simulink model "YXPChFPID_jhua"  (Simulink 5.0)
settings: Solver=ode45  SolverMode=SingleTasking  StartTime=0.0  StopTime=1  FixedStep=0.001  RelTol=1e-3
settings Model: LastModifiedBy=ThinkPad  RTWOptions="-aEnforceIntegerDowncast=1 -aExtMode=0 -aExtModeTesting=0 -aFoldNonRolledExpr=1 -aForceParamTrailComments=0 -aGenerateComments=1 -aGenerateReport=0 -aIgnoreCustomStorageClasses=1 -aIncDataTypeInIds=0 -aIncHierarchyInIds=0 -aInlineInvariantSignals=0 -aInlinedPrmAccess=\"Literals\" -aLocalBlockOutputs=1 -aLogVarNameModifier=\"rt_\" -aMaxRTWIdLen=31 -aPrefixModelToSubsysFcnNames=1 -aRTWVerbose=1 -aRollThreshold=5 -aShowEliminatedStatements=0"

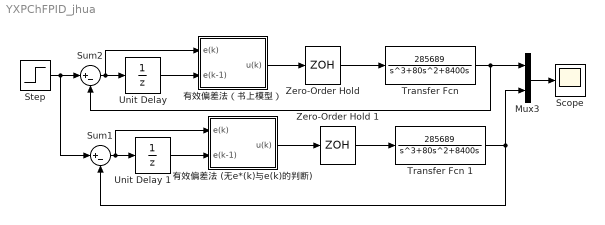
== system YXPChFPID_jhua ==
  "  Scope " : Scope
      settings: YMin=0  YMax=1.8  SaveName=YXPChFPIDI1  DataFormat=Array  MaxDataPoints=500000
  " Transfer Fcn " : TransferFcn  Numerator=[285689]  Denominator=[1 80 8400 0]
  " Transfer Fcn 1" : TransferFcn  Numerator=[285689]  Denominator=[1 80 8400 0]
  " Unit Delay " : UnitDelay  SampleTime=0.001
  " Unit Delay 1" : UnitDelay  SampleTime=0.001
  " Zero-Order Hold " : ZeroOrderHold  SampleTime=0.001
  " Zero-Order Hold 1" : ZeroOrderHold  SampleTime=0.001
  Mux3 : Mux  Inputs=2
  Step : Step  Time=0  After=30  SampleTime=0
  Sum1 : Sum  Inputs=|+-  SaturateOnIntegerOverflow=on
  Sum2 : Sum  Inputs=|+-  SaturateOnIntegerOverflow=on
  有效偏差法 (无e*(k)与e(k)的判断) : Subsystem
  有效偏差法（书上模型） : Subsystem
  wires:
  Step/1 -> Sum2/1, Sum1/1
  有效偏差法（书上模型）/1(u(k)) -> " Zero-Order Hold "/1
  " Zero-Order Hold "/1 -> " Transfer Fcn "/1
  " Transfer Fcn "/1 -> Sum2/2, Mux3/1
  " Unit Delay "/1 -> 有效偏差法（书上模型）/2(e(k-1))
  Sum2/1 -> " Unit Delay "/1, 有效偏差法（书上模型）/1(e(k))
  Mux3/1 -> "  Scope "/1
  有效偏差法 (无e*(k)与e(k)的判断)/1(u(k)) -> " Zero-Order Hold 1"/1
  " Zero-Order Hold 1"/1 -> " Transfer Fcn 1"/1
  " Unit Delay 1"/1 -> 有效偏差法 (无e*(k)与e(k)的判断)/2(e(k-1))
  Sum1/1 -> 有效偏差法 (无e*(k)与e(k)的判断)/1(e(k)), " Unit Delay 1"/1
  " Transfer Fcn 1"/1 -> Mux3/2, Sum1/2

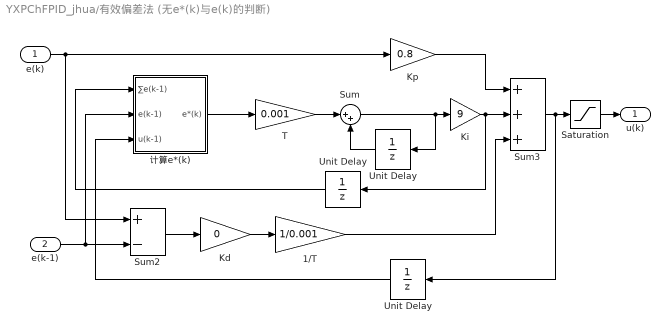
== system YXPChFPID_jhua/有效偏差法 (无e*(k)与e(k)的判断) ==
  e(k) : Inport
  e(k-1) : Inport  Port=2
  " Unit Delay " : UnitDelay  Orientation=left  SampleTime=0.001
  1/T : Gain  Gain=1/0.001  SaturateOnIntegerOverflow=on
  Kd : Gain  Gain=0  SaturateOnIntegerOverflow=on
  Ki : Gain  Gain=9  SaturateOnIntegerOverflow=on
  Kp : Gain  Gain=0.8  SaturateOnIntegerOverflow=on
  Saturation : Saturate  UpperLimit=10  LowerLimit=-10
  Sum : Sum  Inputs=|++  SaturateOnIntegerOverflow=on
  Sum2 : Sum  Inputs=+-  SaturateOnIntegerOverflow=on
  Sum3 : Sum  Inputs=+++  SaturateOnIntegerOverflow=on
  T : Gain  Gain=0.001  SaturateOnIntegerOverflow=on
  Unit Delay : UnitDelay  Orientation=left  SampleTime=0.001
  "Unit Delay " : UnitDelay  Orientation=left  SampleTime=0.001
  计算e*(k) : Subsystem
  u(k) : Outport
  wires:
  "Unit Delay "/1 -> 计算e*(k)/3(u(k-1))
  T/1 -> Sum/1
  Unit Delay/1 -> Sum/2
  Sum/1 -> Ki/1, Unit Delay/1
  " Unit Delay "/1 -> 计算e*(k)/1(∑e(k-1))
  计算e*(k)/1(e*(k)) -> T/1
  Ki/1 -> " Unit Delay "/1, Sum3/2
  1/T/1 -> Sum3/3
  e(k-1)/1 -> 计算e*(k)/2(e(k-1)), Sum2/2
  Kd/1 -> 1/T/1
  Sum3/1 -> "Unit Delay "/1, Saturation/1
  Kp/1 -> Sum3/1
  e(k)/1 -> Sum2/1, Kp/1
  Sum2/1 -> Kd/1
  Saturation/1 -> u(k)/1

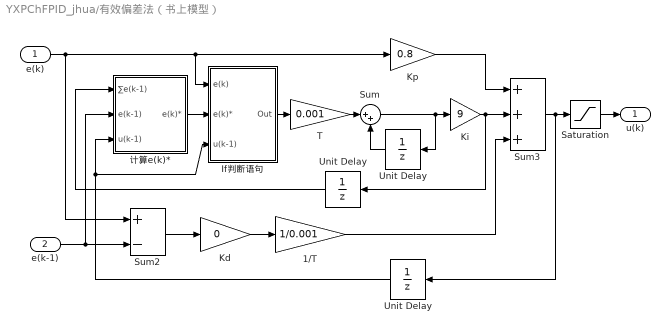
== system YXPChFPID_jhua/有效偏差法（书上模型） ==
  e(k) : Inport
  e(k-1) : Inport  Port=2
  " Unit Delay " : UnitDelay  Orientation=left  SampleTime=0.001
  1/T : Gain  Gain=1/0.001  SaturateOnIntegerOverflow=on
  If判断语句 : Subsystem
  Kd : Gain  Gain=0  SaturateOnIntegerOverflow=on
  Ki : Gain  Gain=9  SaturateOnIntegerOverflow=on
  Kp : Gain  Gain=0.8  SaturateOnIntegerOverflow=on
  Saturation : Saturate  UpperLimit=10  LowerLimit=-10
  Sum : Sum  Inputs=|++  SaturateOnIntegerOverflow=on
  Sum2 : Sum  Inputs=+-  SaturateOnIntegerOverflow=on
  Sum3 : Sum  Inputs=+++  SaturateOnIntegerOverflow=on
  T : Gain  Gain=0.001  SaturateOnIntegerOverflow=on
  Unit Delay : UnitDelay  Orientation=left  SampleTime=0.001
  "Unit Delay " : UnitDelay  Orientation=left  SampleTime=0.001
  计算e(k)* : Subsystem
  u(k) : Outport
  wires:
  Saturation/1 -> u(k)/1
  Sum2/1 -> Kd/1
  e(k)/1 -> If判断语句/1(e(k)), Kp/1, Sum2/1
  Kp/1 -> Sum3/1
  Sum3/1 -> Saturation/1, "Unit Delay "/1
  Kd/1 -> 1/T/1
  e(k-1)/1 -> Sum2/2, 计算e(k)*/2(e(k-1))
  1/T/1 -> Sum3/3
  Ki/1 -> Sum3/2, " Unit Delay "/1
  计算e(k)*/1(e(k)*) -> If判断语句/2("e(k)* ")
  " Unit Delay "/1 -> 计算e(k)*/1(∑e(k-1))
  If判断语句/1("Out ") -> T/1
  Sum/1 -> Unit Delay/1, Ki/1
  Unit Delay/1 -> Sum/2
  T/1 -> Sum/1
  "Unit Delay "/1 -> 计算e(k)*/3(u(k-1)), If判断语句/3(u(k-1))

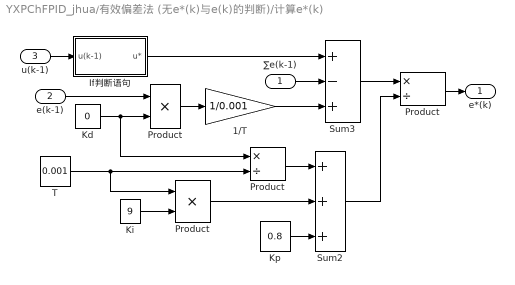
== system YXPChFPID_jhua/有效偏差法 (无e*(k)与e(k)的判断)/计算e*(k) ==
  ∑e(k-1) : Inport
  e(k-1) : Inport  Port=2
  u(k-1) : Inport  Port=3
  " Product" : Product  SaturateOnIntegerOverflow=on
  " Product " : Product  Inputs=*/  SaturateOnIntegerOverflow=on
  1/T : Gain  Gain=1/0.001  SaturateOnIntegerOverflow=on
  If判断语句 : Subsystem
  Kd : Constant  Value=0
  Ki : Constant  Value=9
  Kp : Constant  Value=0.8
  Product : Product  Inputs=*/  SaturateOnIntegerOverflow=on
  "Product " : Product  SaturateOnIntegerOverflow=on
  Sum2 : Sum  Inputs=+++  SaturateOnIntegerOverflow=on
  Sum3 : Sum  Inputs=+-+  SaturateOnIntegerOverflow=on
  T : Constant  Value=0.001
  e*(k) : Outport
  wires:
  If判断语句/1("u* ") -> Sum3/1
  ∑e(k-1)/1 -> Sum3/2
  u(k-1)/1 -> If判断语句/1(u(k-1))
  Product/1 -> e*(k)/1
  Sum2/1 -> Product/2
  Kp/1 -> Sum2/3
  " Product"/1 -> Sum2/2
  " Product "/1 -> Sum2/1
  T/1 -> " Product "/2, " Product"/1
  Kd/1 -> " Product "/1, "Product "/2
  Sum3/1 -> Product/1
  1/T/1 -> Sum3/3
  e(k-1)/1 -> "Product "/1
  "Product "/1 -> 1/T/1
  Ki/1 -> " Product"/2

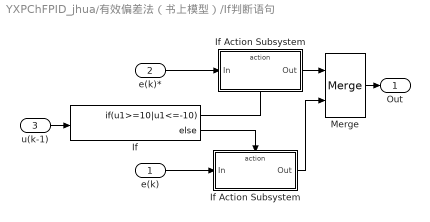
== system YXPChFPID_jhua/有效偏差法（书上模型）/If判断语句 ==
  e(k) : Inport
  "e(k)* " : Inport  Port=2
  u(k-1) : Inport  Port=3
  If : If  IfExpression=u1>=10|u1<=-10
  If Action Subsystem : Subsystem  TreatAsAtomicUnit=on
  "If Action Subsystem " : Subsystem  TreatAsAtomicUnit=on
  Merge : Merge
  "Out " : Outport
  wires:
  If/2 -> "If Action Subsystem "/Action
  e(k)/1 -> "If Action Subsystem "/1("In ")
  u(k-1)/1 -> If/1
  "If Action Subsystem "/1("Out ") -> Merge/2
  If Action Subsystem/1("Out ") -> Merge/1
  "e(k)* "/1 -> If Action Subsystem/1("In ")
  If/1 -> If Action Subsystem/Action
  Merge/1 -> "Out "/1

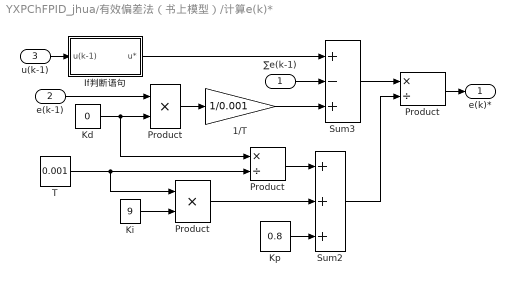
== system YXPChFPID_jhua/有效偏差法（书上模型）/计算e(k)* ==
  ∑e(k-1) : Inport
  e(k-1) : Inport  Port=2
  u(k-1) : Inport  Port=3
  " Product" : Product  SaturateOnIntegerOverflow=on
  " Product " : Product  Inputs=*/  SaturateOnIntegerOverflow=on
  1/T : Gain  Gain=1/0.001  SaturateOnIntegerOverflow=on
  If判断语句 : Subsystem
  Kd : Constant  Value=0
  Ki : Constant  Value=9
  Kp : Constant  Value=0.8
  Product : Product  Inputs=*/  SaturateOnIntegerOverflow=on
  "Product " : Product  SaturateOnIntegerOverflow=on
  Sum2 : Sum  Inputs=+++  SaturateOnIntegerOverflow=on
  Sum3 : Sum  Inputs=+-+  SaturateOnIntegerOverflow=on
  T : Constant  Value=0.001
  e(k)* : Outport
  wires:
  Ki/1 -> " Product"/2
  "Product "/1 -> 1/T/1
  e(k-1)/1 -> "Product "/1
  1/T/1 -> Sum3/3
  Sum3/1 -> Product/1
  Kd/1 -> "Product "/2, " Product "/1
  T/1 -> " Product"/1, " Product "/2
  " Product "/1 -> Sum2/1
  " Product"/1 -> Sum2/2
  Kp/1 -> Sum2/3
  Sum2/1 -> Product/2
  Product/1 -> e(k)*/1
  u(k-1)/1 -> If判断语句/1(u(k-1))
  ∑e(k-1)/1 -> Sum3/2
  If判断语句/1("u* ") -> Sum3/1

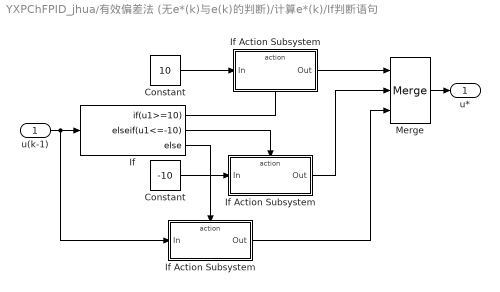
== system YXPChFPID_jhua/有效偏差法 (无e*(k)与e(k)的判断)/计算e*(k)/If判断语句 ==
  u(k-1) : Inport
  Constant : Constant  Value=-10
  "Constant " : Constant  Value=10
  If : If  IfExpression=u1>=10  ElseIfExpressions=u1<=-10
  If Action Subsystem : Subsystem  TreatAsAtomicUnit=on
  "If Action Subsystem " : Subsystem  TreatAsAtomicUnit=on
  "If Action Subsystem  " : Subsystem  TreatAsAtomicUnit=on
  Merge : Merge  Inputs=3
  "u* " : Outport
  wires:
  "If Action Subsystem "/1("Out ") -> Merge/3
  If/3 -> "If Action Subsystem "/Action
  If/2 -> "If Action Subsystem  "/Action
  Merge/1 -> "u* "/1
  If/1 -> If Action Subsystem/Action
  "Constant "/1 -> If Action Subsystem/1("In ")
  If Action Subsystem/1("Out ") -> Merge/1
  "If Action Subsystem  "/1("Out ") -> Merge/2
  u(k-1)/1 -> "If Action Subsystem "/1("In "), If/1
  Constant/1 -> "If Action Subsystem  "/1("In ")

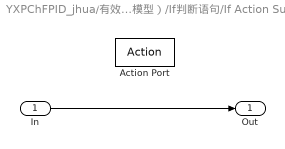
== system YXPChFPID_jhua/有效偏差法（书上模型）/If判断语句/If Action Subsystem ==
  "In " : Inport
  Action Port : ActionPort  ActionType=then
  "Out " : Outport
  wires:
  "In "/1 -> "Out "/1

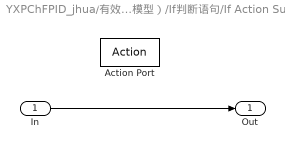
== system YXPChFPID_jhua/有效偏差法（书上模型）/If判断语句/If Action Subsystem  ==
  "In " : Inport
  Action Port : ActionPort  ActionType=else
  "Out " : Outport
  wires:
  "In "/1 -> "Out "/1

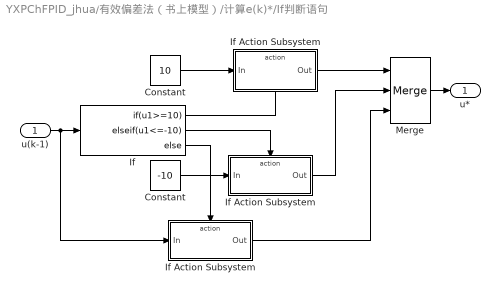
== system YXPChFPID_jhua/有效偏差法（书上模型）/计算e(k)*/If判断语句 ==
  u(k-1) : Inport
  Constant : Constant  Value=-10
  "Constant " : Constant  Value=10
  If : If  IfExpression=u1>=10  ElseIfExpressions=u1<=-10
  If Action Subsystem : Subsystem  TreatAsAtomicUnit=on
  "If Action Subsystem " : Subsystem  TreatAsAtomicUnit=on
  "If Action Subsystem  " : Subsystem  TreatAsAtomicUnit=on
  Merge : Merge  Inputs=3
  "u* " : Outport
  wires:
  Constant/1 -> "If Action Subsystem  "/1("In ")
  u(k-1)/1 -> If/1, "If Action Subsystem "/1("In ")
  "If Action Subsystem  "/1("Out ") -> Merge/2
  If Action Subsystem/1("Out ") -> Merge/1
  "Constant "/1 -> If Action Subsystem/1("In ")
  If/1 -> If Action Subsystem/Action
  Merge/1 -> "u* "/1
  If/2 -> "If Action Subsystem  "/Action
  If/3 -> "If Action Subsystem "/Action
  "If Action Subsystem "/1("Out ") -> Merge/3

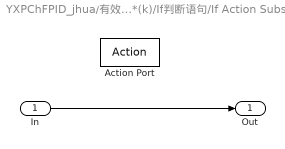
== system YXPChFPID_jhua/有效偏差法 (无e*(k)与e(k)的判断)/计算e*(k)/If判断语句/If Action Subsystem ==
  "In " : Inport
  Action Port : ActionPort  ActionType=then
  "Out " : Outport
  wires:
  "In "/1 -> "Out "/1

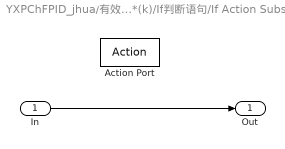
== system YXPChFPID_jhua/有效偏差法 (无e*(k)与e(k)的判断)/计算e*(k)/If判断语句/If Action Subsystem  ==
  "In " : Inport
  Action Port : ActionPort  ActionType=else
  "Out " : Outport
  wires:
  "In "/1 -> "Out "/1

== system YXPChFPID_jhua/有效偏差法 (无e*(k)与e(k)的判断)/计算e*(k)/If判断语句/If Action Subsystem   ==
  "In " : Inport
  Action Port : ActionPort  ActionType=elseif
  "Out " : Outport
  wires:
  "In "/1 -> "Out "/1

== system YXPChFPID_jhua/有效偏差法（书上模型）/计算e(k)*/If判断语句/If Action Subsystem ==
  "In " : Inport
  Action Port : ActionPort  ActionType=then
  "Out " : Outport
  wires:
  "In "/1 -> "Out "/1

== system YXPChFPID_jhua/有效偏差法（书上模型）/计算e(k)*/If判断语句/If Action Subsystem  ==
  "In " : Inport
  Action Port : ActionPort  ActionType=else
  "Out " : Outport
  wires:
  "In "/1 -> "Out "/1

== system YXPChFPID_jhua/有效偏差法（书上模型）/计算e(k)*/If判断语句/If Action Subsystem   ==
  "In " : Inport
  Action Port : ActionPort  ActionType=elseif
  "Out " : Outport
  wires:
  "In "/1 -> "Out "/1
